simulink model "simulink_falcon"  (R2023a)
settings: Solver=VariableStepAuto  StartTime=0.0  StopTime=10.0  RelTol=1e-3
values from neighbouring files (symbols this model uses):
  A1 = 0.3    [matlab_file.m]
  A2 = 2    [matlab_file.m]
  Cd1 = .04    (= 0.04)    [matlab_file.m]
  Cd2 = 0.3    [matlab_file.m]
  g = 9.81    [matlab_file.m]
  m = 1    [matlab_file.m]
  rho = 1.293    [matlab_file.m]
settings Model: Creator=miste  LastModifiedBy=miste

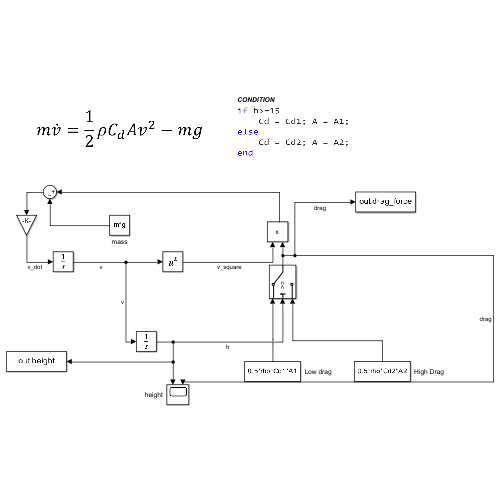
[thumbnail: Simulink's stored preview of the top-level diagram]
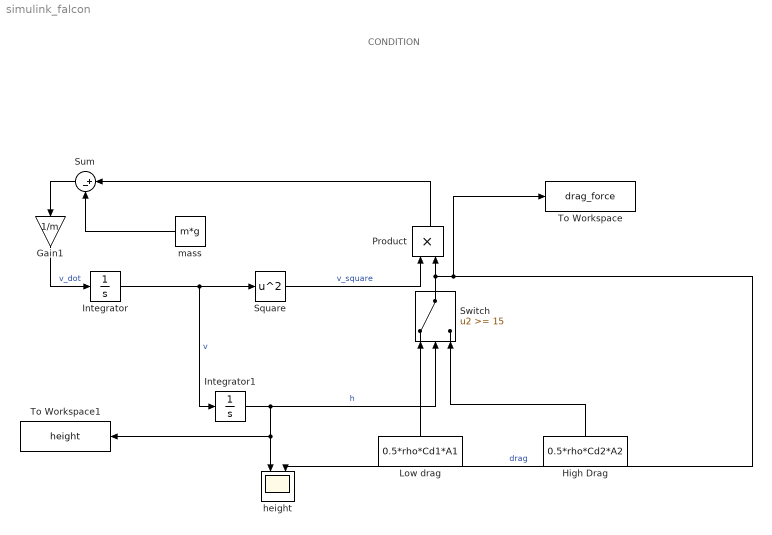
== system simulink_falcon ==
  note: CONDITION
  Gain1 : Gain  Gain=1/m
  High Drag : Constant  Value=0.5*rho*Cd2*A2  VectorParams1D=off
  Integrator : Integrator
  Integrator1 : Integrator  InitialCondition=200
  Low drag : Constant  Value=0.5*rho*Cd1*A1  VectorParams1D=off
  Product : Product
  Square : Math  Operator=square
  Sum : Sum  Inputs=|+-
  Switch : Switch  Threshold=15  SaturateOnIntegerOverflow=off  InputSameDT=off
  To Workspace : ToWorkspace  VariableName=drag_force  SaveFormat=Timeseries  SampleTime=-1
  To Workspace1 : ToWorkspace  VariableName=height  SaveFormat=Timeseries  SampleTime=-1
  height : Scope  NumInputPorts=2
  mass : Constant  Value=m*g
  wires:
  Integrator/1 -> Integrator1/1, Square/1  "v"
  Square/1 -> Product/1  "v_square"
  Product/1 -> Sum/1
  mass/1 -> Sum/2
  Gain1/1 -> Integrator/1  "v_dot"
  Sum/1 -> Gain1/1
  Integrator1/1 -> Switch/2, height/1, To Workspace1/1  "h"
  Switch/1 -> To Workspace/1, height/2, Product/2  "drag"
  Low drag/1 -> Switch/1
  High Drag/1 -> Switch/3
